simulink library "motohawk_engine_motoshare_lib"  (Simulink 6.3)
undefined symbols (not defined in the file or in its folder): cast_val, IndPowerMax, lookup_group, motohawk_tex, motohawk_vardec_config_group, motohawk_vardec_path, SampleTime, SteadyStateECT, txtTitle, WarmUpTimeConst
libraries: MotoHawk_lib x211, motohawk_control_primitives_lib x20, motohawk_annotations_lib x7, motohawk_engine_lib x5, AutoDoc_lib x4, motohawk_control_primitives_lib_new x3, motohawk_control_primitives_motoshare_lib x2
(part 1 of 7)
settings Model: Creator=Blake Suhre  LastModifiedBy=Jason_Tartt  StrictBusMsg=None

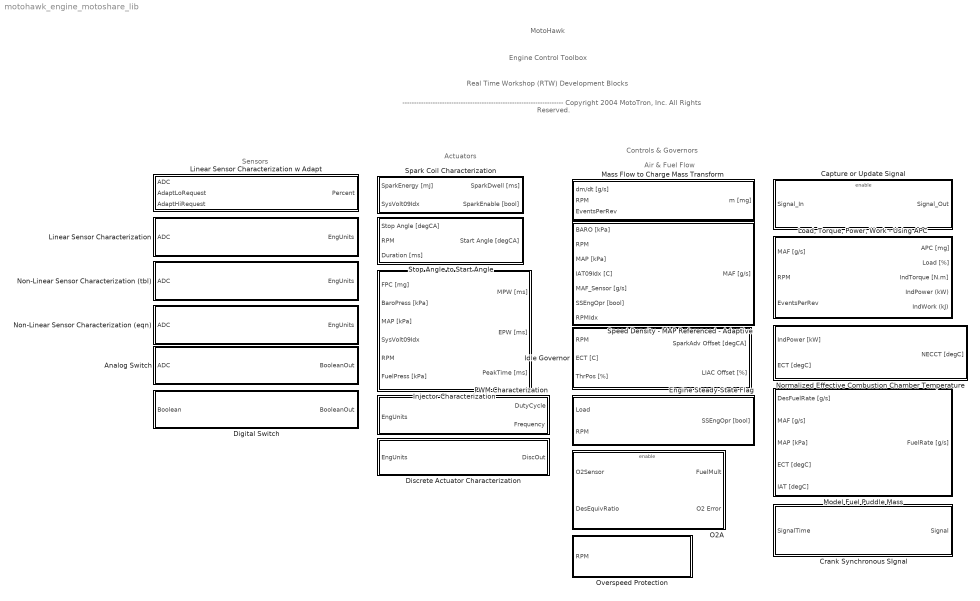
== system motohawk_engine_motoshare_lib ==
  note: Sensors
  note: MotoHawk
  note: ---------------------------------------------------------------------
      | Copyright 2004 MotoTron, Inc.  All Rights Reserved.
  note: Real Time Workshop (RTW)
      | Development Blocks
  note: Engine Control Toolbox
  note: Actuators
  note: Air & Fuel Flow
  note: Controls & Governors
  Analog Switch : Subsystem  mask(Analog Switch Characterization){prefix='ACRequest', nam='ACRequest', units='bool', polarity=High-True, parent_group='Sensors'}
      mask prompts: nam "Name"; parent_group "MotoTune Group"
      mask help:
      | This characterization block is used when digital switch behavior is used on an anolg input pin on the module.  This block inludes a calibratable threshold on the input ADC to convert that signal into a boolean signal.
      |
      | There are additional provisions to calibrate the polarity of the input and apply de-bounce delays to the switching.
      mask init:
      | lbl = ['Analog Switch: ' nam ' [' units ']'];
      | group = [parent_group ' | ' nam];
      mask StyleString: edit,edit,edit,popup(High-True|Low-True),edit
      mask Display:
      | patch([0 0 1 1], [0 0.075 0.075 0], [230/255 0/255 0/255])
      | patch([0 0 1 1], [0.025 0.05 0.05 0.025], [150/255 0/255 0/255])
      | patch([0 0 1 1], [0 0.025 0.025 0], [0/255 0/255 0/255])
      | 
      | disp(lbl);
  Capture or Update Signal : Subsystem  mask(Capture Signal At Startup){nam='Baro', count=5, units='kPa', grp='Engine Control | Run | Airflow'}
      mask prompts: nam "Signal Name"; count "Number Of Samples To Average"; grp "MotoTune GroupString Name"
      mask init:
      | lbl = sprintf('LATCH SIGNAL\nAverage of %d Samples', count);
      mask Display:
      | patch([0 0 1 1], [0 0.075 0.075 0], [230/255 0/255 0/255])
      | patch([0 0 1 1], [0.025 0.05 0.05 0.025], [150/255 0/255 0/255])
      | patch([0 0 1 1], [0 0.025 0.025 0], [0/255 0/255 0/255])
      | 
      | disp(lbl);
  Crank Synchronous SIgnal : Subsystem
      mask Type: Crank Based Sensor Value
      mask Description: This subsystem averages input signal captured at 0 and 360 degrees.
      mask Display:
      | patch([0 0 1 1], [0 0.075 0.075 0], [230/255 0/255 0/255])
      | patch([0 0 1 1], [0.025 0.05 0.05 0.025], [150/255 0/255 0/255])
      | patch([0 0 1 1], [0 0.025 0.025 0], [0/255 0/255 0/255])
      | 
      | disp('CRANK SYNCHRONOUS \nSIGNAL')
  Digital Switch : Subsystem  mask(Digital Switch Characterization){prefix='BrakeRequest', nam='BrakeRequest', units='bool', polarity=High-True, parent_group='Sensors'}
      mask prompts: nam "Name"; parent_group "MotoTune Group"
      mask help:
      | This characterization block is used when digital switch behavior is used on a digital input pin on the module.
      |
      | There are additional provisions to calibrate the polarity of the input and apply de-bounce delays to the switching.
      mask init:
      | lbl = ['Digital Switch: ' nam ' [' units ']'];
      | group = [parent_group ' | ' nam];
      mask StyleString: edit,edit,edit,popup(High-True|Low-True),edit
      mask Display:
      | patch([0 0 1 1], [0 0.075 0.075 0], [230/255 0/255 0/255])
      | patch([0 0 1 1], [0.025 0.05 0.05 0.025], [150/255 0/255 0/255])
      | patch([0 0 1 1], [0 0.025 0.025 0], [0/255 0/255 0/255])
      | 
      | disp(lbl);
  Discrete Actuator Characterization : Subsystem  mask(Discrete Actuator Characterization){prefix='MIL', nam='MIL', units='bool', parent_group='Actuators', polarity=High-True}
      mask prompts: nam "Name"; parent_group "MotoTune Group"
      mask help: Provides the ability to calibrate the polarity of the output digital state before it is applied to the digital output pin.
      mask init:
      | lbl = ['Discrete Characterization:  ' nam ];
      | group = [parent_group ' | ' nam];
      mask StyleString: edit,edit,edit,edit,popup(High-True|Low-True)
      mask Display:
      | patch([0 0 1 1], [0 0.075 0.075 0], [230/255 0/255 0/255])
      | patch([0 0 1 1], [0.025 0.05 0.05 0.025], [150/255 0/255 0/255])
      | patch([0 0 1 1], [0 0.025 0.025 0], [0/255 0/255 0/255])
      | 
      | disp(lbl);
  Engine Steady-State Flag : Subsystem  Description=|  mask(Steady-State Engine Operation){samp_time=SampleTime, group='Engine Control | States | States Config'}
      | /* Name: SSTorqueFilterConst Unit:sec ClassID:VAR StorageID:FLASH Access:RW4+RW3+NA2+NA1 TypeID:UINT2            
      |    Gain:0.001 Min:0.00 Max:65.54 Format:4.2 UpdateID:REMOTE Group:"Engine Control | States" Help:"First-order "  
      |    "filter time constant used to filter torque. This value must be less than SSTorqueTol from unfiltered torque "
      |    "before the steady-state flag can be enabled." VardecSig:6C */                                                
      |                                                                                                                  
      | /* Name: SSRPMFilterConst Unit:sec ClassID:VAR StorageID:FLASH Access:RW4+RW3+NA2+NA1 TypeID:UINT2               
      |    Gain:0.001 Min:0.00 Max:65.54 Format:4.2 UpdateID:REMOTE Group:"Engine Control | States" Help:"First-order "  
      |    "filter time constant used to filter torque. This value must be less than SSRPMTol from unfiltered torque "   
      |    "before the steady-state flag can be enabled." VardecSig:6C */                                                
      |                                                                                                                  
      | /* Name: SSTorqueTol Unit:N.m ClassID:VAR StorageID:FLASH Access:RW4+RW3+NA2+NA1 TypeID:UINT2 Gain:0.001         
      |    Min:0.00 Max:65.54 Format:4.2 UpdateID:REMOTE Group:"Engine Control | States" Help:"Tolerance within which "  
      |    "the difference between filtered and unfiltered torque must lie before the steady-state flag can be "         
      |    "enabled." VardecSig:6C */                                                                                    
      |                                                                                                                  
      | /* Name: SSRPMTol Unit:RPM ClassID:VAR StorageID:FLASH Access:RW4+RW3+NA2+NA1 TypeID:UINT2 Gain:0.01             
      |    Min:0.00 Max:655.35 Format:4.2 UpdateID:REMOTE Group:"Engine Control | States" Help:"Tolerance within which " 
      |    "the difference between filtered and unfiltered RPM must lie before the steady-state flag can be enabled."    
      |    VardecSig:6C */
      mask prompts: samp_time "Sample Time [s]:"; group "MotoTune Group String"
      mask help:
      | This block determines whether or not the engine has achieved steady-state operation. It accomplishes this by applying a first-order low-pass filter to the indicated torque and RPM inputs. The filetrcoeficeints are individually calibratable for each. Once both the filtered torque and RPM values are within the calibratable toleraance of the input values, engine operation is assumed to be steady-state.
      |
      | If 'Sample Time' is -1, then extra code and RAM will be generated to dynamically calculate dt.
      mask Display:
      | patch([0 0 1 1], [0 0.075 0.075 0], [230/255 0/255 0/255])
      | patch([0 0 1 1], [0.025 0.05 0.05 0.025], [150/255 0/255 0/255])
      | patch([0 0 1 1], [0 0.025 0.025 0], [0/255 0/255 0/255])
      | 
      | disp('ENGINE\nSTEADY-STATE\nDETERMINATION')
  Idle Governor : Subsystem
      mask Display:
      | patch([0 0 1 1], 0.5*[0 0.075 0.075 0], [230/255 0/255 0/255])
      | patch([0 0 1 1], 0.5*[0.025 0.05 0.05 0.025], [150/255 0/255 0/255])
      | patch([0 0 1 1], 0.5*[0 0.025 0.025 0], [0/255 0/255 0/255])
      | 
      | disp('IDLE GOVERNOR');
  Injector Characterization : Subsystem  Description=|
      | /* Name: InjGain Unit:ms/mg ClassID:VAR StorageID:FLASH Access:RW4+RW3+NA2+NA1 TypeID:UINT2 Gain:0.0001       
      |    Min:0.0000 Max:6.5500 Format:5.4 UpdateID:REMOTE Group:"Actuators | Injectors | Config" Help:"Gain valued "
      |    "used in the linear transformation of FPC to mechanical pulsewidth." VardecSig:6C */                       
      |                                                                                                               
      | /* Name: InjOfst Unit:ms ClassID:VAR StorageID:FLASH Access:RW4+RW3+NA2+NA1 TypeID:SINT2 Gain:0.0001          
      |    Min:-3.2768 Max:3.2767 Format:5.4 UpdateID:REMOTE Group:"Actuators | Injectors | Config" Help:"Offset "    
      |    "valued used in the linear transformation of FPC to mechanical pulsewidth." VardecSig:6C */                
      |                                                                                                               
      | /* Name: SysVolt10IdxArr Unit:volt ClassID:ORDARR StorageID:FLASH Access:RW4+RW3+NA2+NA1 TypeID:UINT1         
      |    Gain:0.1 Min:0.00 Max:25.50 Format:4.2 UpdateID:REMOTE OrdLen:10 Group:"Global Index Arrays | Voltage"     
      |    Help:"Ten breakpoint system voltage index array." VardecSig:6C */                                          
      |                                                                                                               
      | /* Name: InjTurnOnTbl Unit:ms ClassID:TBL StorageID:FLASH Access:RW4+RW3+NA2+NA1 TypeID:UINT2 Gain:0.001      
      |    Min:0.0000 Max:65.5350 Format:5.4 UpdateID:REMOTE OrdArr:SysVolt10IdxArr Group:"Actuators | Injectors"     
      |    Help:"Injector turn on time as a function of system voltage." VardecSig:6C */                              
      |                                                                                                               
      | /* Name: InjDeltaPress10IdxArr Unit:kPa ClassID:ORDARR StorageID:FLASH Access:RW4+RW3+NA2+NA1 TypeID:UINT2    
      |    Gain:0.1 Min:0.0 Max:6553.0 Format:5.1 UpdateID:REMOTE OrdLen:10 Group:"Actuators | Injectors" Help:"Ten " 
      |    "breakpoint fuel delta pressure index array." VardecSig:6C */                                              
      |                                                                                                               
      | /* Name: FueldPCompTbl Unit:kPa ClassID:TBL StorageID:FLASH Access:RW4+RW3+NA2+NA1 TypeID:UINT2 Gain:0.1      
      |    Min:0.0 Max:6553.0 Format:5.1 UpdateID:REMOTE OrdArr:InjDeltaPress10IdxArr Group:"Actuators | Injectors"   
      |    Help:"Injector delta pressure compensation table." VardecSig:6C */                                         
      |                                                                                                               
      | /* Name: InjTurnOffTbl Unit:ms ClassID:TBL StorageID:FLASH Access:RW4+RW3+NA2+NA1 TypeID:UINT2                
      |    Gain:0.01 Min:0.00 Max:655.00 Format:5.2 UpdateID:REMOTE OrdArr:InjDeltaPress10IdxArr Group:"Actuators | " 
      |    "Injectors" Help:"Injector turn off time table." VardecSig:6C */                                           
      |                                                                                                               
      | /* Name: InjMPW Unit:ms ClassID:VAR StorageID:RAM Access:RO4+RO3+NA2+NA1 TypeID:UINT2 Gain:0.01 Min:0.00      
      |    Max:655.35 Format:5.2 UpdateID:BACKGND Group:"Actuators | Injectors" Help:"Injector mechanical pulse "     
      |    "width." VardecSig:6C */                                                                                   
      |                                                                                                               
      | /* Name: InjEPW Unit:ms ClassID:VAR StorageID:RAM Access:RO4+RO3+NA2+NA1 TypeID:UINT2 Gain:0.01 Min:0.00      
      |    Max:655.35 Format:5.2 UpdateID:BACKGND Group:"Actuators | Injectors" Help:"Injector electrical pulse "     
      |    "width." VardecSig:6C */                                                                                   
      |                                                                                                               
      | /* Name: InjDeltaPress Unit:kPa ClassID:VAR StorageID:RAM Access:RO4+RO3+NA2+NA1 TypeID:UINT2 Gain:0.01       
      |    Min:0.00 Max:655.35 Format:5.2 UpdateID:BACKGND Group:"Actuators | Injectors" Help:"Delta pressure across "
      |    "the injector." VardecSig:6C */                                                                            
      | /* Name: FuelFlowCompMap Unit:mult ClassID:MAP StorageID:RAM Access:RO4+RO3+NA2+NA1 TypeID:UINT2              
      |    Gain:0.0001 Min:0.0000 Max:2.0000 Format:5.4 UpdateID:BACKGND XOrdArr:IndTorque10IdxArr YOrdArr:RPM10IdxArr
      |    Group:"Actuators | Injectors" Help:"Correction for injector fuel flow differences between injector test "  
      |    "bench and engine operating in the conditions. This map should only be calibrated after volumetric "       
      |    "efficiency has been calibrated to a reference airflow measurement device." VardecSig:6C */
      mask Description: Injector characterization block.
      mask Help: Converts the calculated fuel charge mass (FPC) value to the required electrical pulsewidth. Requires gain, offset, turn-on time vs. voltage, turn-off time vs. injector delta pressure and delta pressure pulsewidth compensation. A choice of five different injector delta pressure calculation methods are offered.
      mask Display:
      | patch([0 0 1 1], [0 0.075 0.075 0], [230/255 0/255 0/255])
      | patch([0 0 1 1], [0.025 0.05 0.05 0.025], [150/255 0/255 0/255])
      | patch([0 0 1 1], [0 0.025 0.025 0], [0/255 0/255 0/255])
      | 
      | disp('Injector\nCharacterization')
  Linear Sensor Characterization : Subsystem  mask(Linear Sensor Characterization){nam='MAP', prefix='MAP', units='kPa', inputunits=ADC, samp_time=SampleTime, parent_group='Sensors'}
      mask prompts: nam "Name"; units "Output Units"; inputunits "Input Units"; samp_time "Sample Time"; parent_group "MotoTune Group"
      mask help:
      | Converts from A/D Counts to Engineering Units, using a Gain and Offset.
      | Saturates the converted value around Min and Max values, and triggers a Fault when out of range.
      mask init:
      | lbl = ['Linear Sensor: ' nam ' [' units ']'];
      | group = [parent_group ' | ' nam];
      settings: RTWSystemCode=Function  RTWFcnNameOpts=Use subsystem name  RTWFileNameOpts=Use function name
      mask Display:
      | patch([0 0 1 1], [0 0.075 0.075 0], [230/255 0/255 0/255])
      | patch([0 0 1 1], [0.025 0.05 0.05 0.025], [150/255 0/255 0/255])
      | patch([0 0 1 1], [0 0.025 0.025 0], [0/255 0/255 0/255])
      | 
      | disp(lbl);
  Linear Sensor Characterization w Adapt : Subsystem  mask(Potentiometer Characterization with adapting endpoints.){nam='TPS', prefix='TPS', samp_time=.005, parent_group='Sensors | TPS'}
      mask prompts: nam "Name"; samp_time "Sample Time"; parent_group "MotoTune Group"
      mask help:
      | This block transforms the input from a potentiometer into a percentage, refering to the percentage of travel within the scale.
      |
      | The endpoints of the scale will adapt based on the values that block sees on the input.
      mask init:
      | lbl = ['Linear Sensor: ' nam ' [%]'];
      | lbl2 = ['With Adaption'];
      | group = [parent_group ' | ' nam];
      | units = '%';
      mask Display:
      | patch([0 0 1 1], [0 0.075 0.075 0], [230/255 0/255 0/255])
      | patch([0 0 1 1], [0.025 0.05 0.05 0.025], [150/255 0/255 0/255])
      | patch([0 0 1 1], [0 0.025 0.025 0], [0/255 0/255 0/255])
      | 
      | 
      | 
      | text(0.6,0.60,lbl,'horizontalAlignment','center');
      | text(0.6,0.30,lbl2,'horizontalAlignment','center');
  "Load, Torque, Power, Work - Using APC" : Subsystem
      mask Display:
      | patch([0 0 1 1], 0.8*[0 0.075 0.075 0], [230/255 0/255 0/255])
      | patch([0 0 1 1], 0.8*[0.025 0.05 0.05 0.025], [150/255 0/255 0/255])
      | patch([0 0 1 1], 0.8*[0 0.025 0.025 0], [0/255 0/255 0/255])
      | 
      | disp('LOAD, TORQUE,\nPOWER, AND WORK\nCOMPUTATION\nUSING APC');
  Mass Flow to Charge Mass Transform : Subsystem
      mask Description: Converts mass flow rate to the equivalent per cylinder charge mass.
      mask Help:
      | Given the mass flow rate [g/s], RPM and the total number of combustion events per crankshaft revolution, this block calculates the equivalent charge mass ingested per cylinder.
      | 
      | Note: as an example, the number of cylinder events per revolution would be 2 for a four cylinder four-stroke engine and 4 for a four-cylinder two-stroke engine.
      mask Display:
      | patch([0 0 1 1], [0 0.075 0.075 0], [230/255 0/255 0/255])
      | patch([0 0 1 1], [0.025 0.05 0.05 0.025], [150/255 0/255 0/255])
      | patch([0 0 1 1], [0 0.025 0.025 0], [0/255 0/255 0/255])
      | 
      | disp('MASS FLOW\nTO CHARGE MASS\nTRANSFORM')
  Model Fuel Puddle Mass : Subsystem  mask{group_cal='Engine Control | Run | Fuel | Transient Fuel', group_dis='Engine Control | Run | Fuel | Transient Fuel'}
      mask prompts: group_cal "MotoTune Calibration Group String"; group_dis "MotoTune Display Group String"
      mask Display:
      | patch([0 0 1 1], 0.5*[0 0.075 0.075 0], [230/255 0/255 0/255])
      | patch([0 0 1 1], 0.5*[0.025 0.05 0.05 0.025], [150/255 0/255 0/255])
      | patch([0 0 1 1], 0.5*[0 0.025 0.025 0], [0/255 0/255 0/255])
      | 
      | disp('TAU-X\nTRANSIENT\nFUELING');
  Non-Linear Sensor Characterization (eqn) : Subsystem  mask(Non-Linear Sensor Characterization (eqn)){nam='ECT', prefix='ECT', units='C', inputunits='ADC', numcoef=6, samp_time=SampleTime, parent_group='Sensors'}
      mask prompts: nam "Name"; units "Output Units"; inputunits "Input Units"; numcoef "Number Of Coefficients"; samp_time "Sample Time"; parent_group "MotoTune Group"
      mask help:
      | Converts from A/D Counts to Engineering Units using a calibration polynomial.
      | Saturates the converted value around Min and Max values and triggers a Fault when out of range.
      mask init:
      | lbl = ['Non-Linear Sensor (eqn): ' nam ' [' units ']'];
      | group = [parent_group ' | ' nam];
      settings: RTWSystemCode=Function  RTWFcnNameOpts=Use subsystem name  RTWFileNameOpts=Use function name
      mask Display:
      | patch([0 0 1 1], [0 0.075 0.075 0], [230/255 0/255 0/255])
      | patch([0 0 1 1], [0.025 0.05 0.05 0.025], [150/255 0/255 0/255])
      | patch([0 0 1 1], [0 0.025 0.025 0], [0/255 0/255 0/255])
      | 
      | disp(lbl);
  Non-Linear Sensor Characterization (tbl) : Subsystem  mask(Non-Linear Sensor Characterization (tbl)){nam='IAT', prefix='IAT', units='C', inputunits='ADC', tblsize=20, samp_time=SampleTime, parent_group='Sensors'}
      mask prompts: nam "Name"; units "Output Units"; inputunits "Input Units"; tblsize "Table Size"; samp_time "Sample Time"; parent_group "MotoTune Group"
      mask help:
      | Converts from A/D Counts to Engineering Units using a 1-D Table Lookup.
      | Saturates the converted value around Min and Max values and triggers a Fault when out of range.
      mask init:
      | lbl = ['Non-Linear Sensor (tbl): ' nam ' [' units ']'];
      | group = [parent_group ' | ' nam];
      settings: RTWSystemCode=Function  RTWFcnNameOpts=Use subsystem name  RTWFileNameOpts=Use function name
      mask Display:
      | patch([0 0 1 1], [0 0.075 0.075 0], [230/255 0/255 0/255])
      | patch([0 0 1 1], [0.025 0.05 0.05 0.025], [150/255 0/255 0/255])
      | patch([0 0 1 1], [0 0.025 0.025 0], [0/255 0/255 0/255])
      | 
      | disp(lbl);
  Normalized Effective Combustion Chamber Temperature : Subsystem  Description=|  mask(Steady-State Engine Operatio){}
      | /* Name: SSTorqueFilterConst Unit:sec ClassID:VAR StorageID:FLASH Access:RW4+RW3+NA2+NA1 TypeID:UINT2            
      |    Gain:0.001 Min:0.00 Max:65.54 Format:4.2 UpdateID:REMOTE Group:"Engine Control | States" Help:"First-order "  
      |    "filter time constant used to filter torque. This value must be less than SSTorqueTol from unfiltered torque "
      |    "before the steady-state flag can be enabled." VardecSig:6C */                                                
      |                                                                                                                  
      | /* Name: SSRPMFilterConst Unit:sec ClassID:VAR StorageID:FLASH Access:RW4+RW3+NA2+NA1 TypeID:UINT2               
      |    Gain:0.001 Min:0.00 Max:65.54 Format:4.2 UpdateID:REMOTE Group:"Engine Control | States" Help:"First-order "  
      |    "filter time constant used to filter torque. This value must be less than SSRPMTol from unfiltered torque "   
      |    "before the steady-state flag can be enabled." VardecSig:6C */                                                
      |                                                                                                                  
      | /* Name: SSTorqueTol Unit:N.m ClassID:VAR StorageID:FLASH Access:RW4+RW3+NA2+NA1 TypeID:UINT2 Gain:0.001         
      |    Min:0.00 Max:65.54 Format:4.2 UpdateID:REMOTE Group:"Engine Control | States" Help:"Tolerance within which "  
      |    "the difference between filtered and unfiltered torque must lie before the steady-state flag can be "         
      |    "enabled." VardecSig:6C */                                                                                    
      |                                                                                                                  
      | /* Name: SSRPMTol Unit:RPM ClassID:VAR StorageID:FLASH Access:RW4+RW3+NA2+NA1 TypeID:UINT2 Gain:0.01             
      |    Min:0.00 Max:655.35 Format:4.2 UpdateID:REMOTE Group:"Engine Control | States" Help:"Tolerance within which " 
      |    "the difference between filtered and unfiltered RPM must lie before the steady-state flag can be enabled."    
      |    VardecSig:6C */
      mask Display:
      | patch([0 0 1 1], [0 0.075 0.075 0], [230/255 0/255 0/255])
      | patch([0 0 1 1], [0.025 0.05 0.05 0.025], [150/255 0/255 0/255])
      | patch([0 0 1 1], [0 0.025 0.025 0], [0/255 0/255 0/255])
      | 
      | disp('COMBUSTION CHAMBER\nTEMPERATURE');
  O2A : Subsystem  TreatAsAtomicUnit=on  mask(Closed-Loop O2 Control){bank=A, display_group=lookup_group(gcb, 'O2Display'), cal_group=lookup_group(gcb, 'O2BankA')}
      mask prompts: display_group "MotoTune Display Group"; cal_group "MotoTune Calibration Group"
      mask StyleString: popup(A|B),edit,edit
      mask Display:
      | patch([0 0 1 1], 0.5*[0 0.075 0.075 0], [230/255 0/255 0/255])
      | patch([0 0 1 1], 0.5*[0.025 0.05 0.05 0.025], [150/255 0/255 0/255])
      | patch([0 0 1 1], 0.5*[0 0.025 0.025 0], [0/255 0/255 0/255])
      | 
      | disp(['O2 Control\nBank ' bank]);
  Overspeed Protection : Subsystem
      mask Description:
      | Block allows for three levels of overspeed rev limits, and will set three fault accordingly.
      | 
      | Soft Overspeed, Medium Overspeed, and Hard Overspeed.
      mask Display:
      | patch([0 0 1 1], 0.5*[0 0.075 0.075 0], [230/255 0/255 0/255])
      | patch([0 0 1 1], 0.5*[0.025 0.05 0.05 0.025], [150/255 0/255 0/255])
      | patch([0 0 1 1], 0.5*[0 0.025 0.025 0], [0/255 0/255 0/255])
      | 
      | disp('RPM LIMITER');
  PWM Characterization : Subsystem  mask(Linear Actuator Characterization){nam='LIAC', prefix='LIAC_', units='%', parent_group=motohawk_vardec_path(gcb)}
      mask prompts: nam "Name"; parent_group "MotoTune Group"
      mask help:
      | Scales the duty cycle of a PWM signal using a Gain and Offset with a calibratable PWM Frequency.
      | Saturates the converted value around Min and Max values, and converts the signal to the appropriate fixed-point format for use with motoHawk PWM blocks.
      mask init:
      | lbl = ['PWM Characterization: ' nam ];
      | group = [parent_group ' | ' nam];
      settings: RTWSystemCode=Function  RTWFcnNameOpts=Use subsystem name  RTWFileNameOpts=Use function name
      mask Display:
      | patch([0 0 1 1], [0 0.075 0.075 0], [230/255 0/255 0/255])
      | patch([0 0 1 1], [0.025 0.05 0.05 0.025], [150/255 0/255 0/255])
      | patch([0 0 1 1], [0 0.025 0.025 0], [0/255 0/255 0/255])
      | 
      | disp(lbl);
  Spark Coil Characterization : Subsystem  Description=|  mask{group='Actuators | Coils'}
      | /* Name: CoilDrvrDlyTime Unit:us ClassID:VAR StorageID:FLASH Access:RW4+RW3+NA2+NA1 TypeID:UINT2 Gain:0.1       
      |    Min:0.00 Max:6553.50 Format:6.2 UpdateID:REMOTE Group:"Actuators | Coils" Help:"Coil driver delay time "     
      |    "between initiation of the EST signal and the initiation of coil dwell." VardecSig:6C */                     
      |                                                                                                                 
      | /* Name: SysVolt10IdxArr Unit:volt ClassID:VAR StorageID:FLASH Access:RW4+RW3+NA2+NA1 TypeID:UINT1 Gain:0.1     
      |    Min:0.00 Max:25.50 Format:4.2 UpdateID:REMOTE Group:"Global Index Arrays | Voltage" Help:"Ten breakpoint "   
      |    "system voltage index array." VardecSig:6C */                                                                
      |                                                                                                                 
      | /* Name: SpkEnergy10IdxArr Unit:volt ClassID:VAR StorageID:FLASH Access:RW4+RW3+NA2+NA1 TypeID:UINT1            
      |    Gain:0.1 Min:0.00 Max:25.50 Format:4.2 UpdateID:REMOTE Group:"Actuators | Coils" Help:"Ten breakpoint spark "
      |    "energy index array." VardecSig:6C */                                                                        
      |                                                                                                                 
      | /* Name: CoilDwellMap Unit:ms ClassID:MAP StorageID:FLASH Access:RW4+RW3+NA2+NA1 TypeID:UINT2 Gain:0.01         
      |    Min:0.00 Max:655.35 Format:4.2 UpdateID:REMOTE XOrdArr:SpkEnergy10IdxArr YOrdArr:SysVolt10IdxArr             
      |    Group:"Actuators | Coils" Help:"Required coil dwell map as a function of system voltage and spark energy."   
      |    VardecSig:6C */
      mask prompts: group "MotoTune Group String"
      mask help: Coil characterization block.
      mask Help: Given the desired spark energy and system voltage, this block determines the required coil dwell period. Requires calibration of the dwell map and the delay time.
      mask Display:
      | patch([0 0 1 1], [0 0.075 0.075 0], [230/255 0/255 0/255])
      | patch([0 0 1 1], [0.025 0.05 0.05 0.025], [150/255 0/255 0/255])
      | patch([0 0 1 1], [0 0.025 0.025 0], [0/255 0/255 0/255])
      | 
      | disp('COIL\nCHRZN.')
  Speed Density - MAP Referenced - Adaptive : Subsystem  Description=|
      | /* Name: PortPressRatio20IdxArr Unit:unitless ClassID:ORDARR StorageID:FLASH Access:RW4+RW3+NA2+NA1              
      |    TypeID:UINT2 Gain:0.0001 Min:0.0000 Max:6.5535 Format:5.4 UpdateID:REMOTE OrdLen:20 Group:"Engine Control | " 
      |    "Run | Airflow" Help:"Port pressure ratio index array. Used for speed-density flow computations." VardecSig:6E
      |    */                                                                                                            
      |                                                                                                                  
      | /* Name: RPM20IdxArr Unit:RPM20IdxArr ClassID:ORDARR StorageID:FLASH Access:RW4+RW3+NA2+NA1                      
      |    TypeID:UINT2 Gain:0.1 Min:0.0 Max:6553.0 Format:5.1 UpdateID:REMOTE OrdLen:20 Group:"Global "                 
      |    "Index Arrays | RPM" Help:"20 breakpoint RPM index array." VardecSig:5E */                                    
      |                                                                                                                  
      | /* Name: VolEffMap Unit:Unitless ClassID:MAP StorageID:FLASH Access:RW4+RW3+NA2+NA1 TypeID:UINT2                 
      |    Gain:0.0001 Min:0.00 Max:6.55 Format:6.2 UpdateID:REMOTE XOrdArr:PortPressRatio20IdxArr                       
      |    YOrdArr:RPM20IdxArr Group:"Engine Control | Run | Airflow" Help:"Engine volumetric efficency "                
      |    "map." VardecSig:61 */                                                                                        
      |                                                                                                                  
      | /* Name: IAT10IdxArr Unit:C ClassID:ORDARR StorageID:FLASH Access:RW4+RW3+NA2+NA1                                
      |    TypeID:SINT2 Gain:0.01 Min:-327.6800 Max:327.6700 Format:5.4 UpdateID:REMOTE OrdLen:10                        
      |    Group:"Engine Control | Run | Airflow" Help:"10 breakpoint intake air temperture index "                      
      |    "array." VardecSig:5C */                                                                                      
      |                                                                                                                  
      | /* Name: VETempCorrTbl ClassID:TBL StorageID:FLASH Access:RW4+RW3+NA2+NA1 TypeID:UINT2 Gain:0.0001 Min:0.00      
      |    Max:6.55 Format:4.2 UpdateID:REMOTE OrdArr:IAT10IdxArr Group:"Engine Control | Run | Airflow"                 
      |    Help:"Volumetric efficiency temperature correction table." VardecSig:6C */                                    
      |                                                                                                                  
      | /* Name: BaroPress10IdxArr Unit:C ClassID:ORDARR StorageID:FLASH Access:RW4+RW3+NA2+NA1                          
      |    TypeID:UINT2 Gain:0.01 Min:0.0000 Max:655.3500 Format:5.4 UpdateID:REMOTE OrdLen:10                           
      |    Group:"Engine Control | Run | Airflow" Help:"10 breakpoint barometric pressure index "                        
      |    "array." VardecSig:5C */                                                                                      
      |                                                                                                                  
      | /* Name: VEBaroCorrTbl ClassID:TBL StorageID:FLASH Access:RW4+RW3+NA2+NA1 TypeID:UINT2 Gain:0.0001 Min:0.00      
      |    Max:6.55 Format:4.2 UpdateID:REMOTE OrdArr:BaroPress10IdxArr Group:"Engine Control | Run | Airflow"           
      |    Help:"Volumetric efficiency barometric pressure correction table." VardecSig:6C */                            
      |                                                                                                                  
      | /* Name: CylSweptVol Unit:cm^3 ClassID:VAR StorageID:FLASH Access:RW4+RW3+NA2+NA1 TypeID:UINT2 Gain:0.1          
      |    Min:0.0 Max:6553.0 Format:5.1 UpdateID:REMOTE Group:"Engine Control | Run | Airflow" Help:"Cylinder swept "   
      |    "volume." VardecSig:6C */                                                                                     
      |                                                                                                                  
      | /* Name: MAFPort Unit:g/s ClassID:VAR StorageID:RAM Access:RO4+RO3+NA2+NA1 TypeID:UINT2 Gain:0.01                
      |    Min:0.00 Max:655.00 Format:5.2 UpdateID:BACKGND Group:"Engine Control | Run | Airflow" Help:"Total "          
      |    "ingested cylinder charge mass flow rate. The sum of all port flows. This values includes any EGR and "       
      |    "Purge mass flows." VardecSig:6A */                                                                           
      |                                                                                                                  
      | /* Name: CombEventsPerRev ClassID:VAR StorageID:FLASH Access:RW4+RW3+NA2+NA1 TypeID:UINT1 Gain:0.5 Min:0.5       
      |    Max:127.0 Format:4.1 UpdateID:REMOTE Group:"Engine Control | Run | Airflow" Help:"Number of conbustion "      
      |    "events per engine revolution. For example, for a four-stroke, eight cylinder engine the value would be 4."   
      |    VardecSig:6C */
      mask Description: Calculates air mass flow rate per cylinder. The estimated mass flow rate is that of the entire mixture: air, EGR and purge.
      mask Help: Given calibrations for the volumetric efficiency map, cylinder swept volume [cm3] and the VE temperature and pressure correction tables, the block calculates the air mass flow rate [g/s] per cylinder, given the barometric and manifold pressures [kPa], the manifold air temperature [C] and RPM.
      mask Display:
      | patch([0 0 1 1], 0.5*[0 0.075 0.075 0], [230/255 0/255 0/255])
      | patch([0 0 1 1], 0.5*[0.025 0.05 0.05 0.025], [150/255 0/255 0/255])
      | patch([0 0 1 1], 0.5*[0 0.025 0.025 0], [0/255 0/255 0/255])
      | 
      | disp('MAP-REFERENCED\nSPEED-DENSITY\nCOMPUTATION\n(adaptive)');
  Stop Angle to Start Angle : Subsystem  Description=|
      | /* Name: CoilDrvrDlyTime Unit:us ClassID:VAR StorageID:FLASH Access:RW4+RW3+NA2+NA1 TypeID:UINT2 Gain:0.1       
      |    Min:0.00 Max:6553.50 Format:6.2 UpdateID:REMOTE Group:"Actuators | Coils" Help:"Coil driver delay time "     
      |    "between initiation of the EST signal and the initiation of coil dwell." VardecSig:6C */                     
      |                                                                                                                 
      | /* Name: SysVolt10IdxArr Unit:volt ClassID:VAR StorageID:FLASH Access:RW4+RW3+NA2+NA1 TypeID:UINT1 Gain:0.1     
      |    Min:0.00 Max:25.50 Format:4.2 UpdateID:REMOTE Group:"Global Index Arrays | Voltage" Help:"Ten breakpoint "   
      |    "system voltage index array." VardecSig:6C */                                                                
      |                                                                                                                 
      | /* Name: SpkEnergy10IdxArr Unit:volt ClassID:VAR StorageID:FLASH Access:RW4+RW3+NA2+NA1 TypeID:UINT1            
      |    Gain:0.1 Min:0.00 Max:25.50 Format:4.2 UpdateID:REMOTE Group:"Actuators | Coils" Help:"Ten breakpoint spark "
      |    "energy index array." VardecSig:6C */                                                                        
      |                                                                                                                 
      | /* Name: CoilDwellMap Unit:ms ClassID:MAP StorageID:FLASH Access:RW4+RW3+NA2+NA1 TypeID:UINT2 Gain:0.01         
      |    Min:0.00 Max:655.35 Format:4.2 UpdateID:REMOTE XOrdArr:SpkEnergy10IdxArr YOrdArr:SysVolt10IdxArr             
      |    Group:"Actuators | Coils" Help:"Required coil dwell map as a function of system voltage and spark energy."   
      |    VardecSig:6C */
      mask Type: Stop Angle to Start Angle
      mask Description: Stop Angle to Start Angle calculation.  Subtracts the duration of a Pulse Width in the angle domain from a given Stop Angle.
      mask Display:
      | patch([0 0 1 1], [0 0.075 0.075 0], [230/255 0/255 0/255])
      | patch([0 0 1 1], [0.025 0.05 0.05 0.025], [150/255 0/255 0/255])
      | patch([0 0 1 1], [0 0.025 0.025 0], [0/255 0/255 0/255])

== system motohawk_engine_motoshare_lib/Analog Switch ==
  ADC : Inport
  0 = No Inversion 1 = Inversion : MotoHawk_lib/Calibration & Probing Blocks/motohawk_calibration  nam=[prefix 'Polarity']  val=boolean(polarity-1)  storage=Calibration  show_more=on  name_source=Use Parameter  data_type=Inherit from 'Default Value'  read_level=1  write_level=1  ovr_cals=on  view_as=Number  enum_struct={'Disabled', 'Enabled'}  vector_style=Wide Row  use_help_units=on  help="'0 = High True    1 = Low True'"  units='bool'  use_header_enum=off  row_header_enum={}  col_header_enum={}  use_min_max=off  min_val=-inf  max_val=inf  use_precision=off  precision=''  gain=1  offset=0  exp=1  use_mototune_group=on  mototune_group=[group ' | ' nam ' | ' nam ' Config']
  Data Type Conversion : DataTypeConversion  SaturateOnIntegerOverflow=on  RndMeth=Zero
  Logical Operator : Logic  Operator=XOR
  Override in Engineering Units : MotoHawk_lib/Calibration & Probing Blocks/motohawk_override_abs  parent_name=nam  show_more=on  name_source=Use Parameter  parent_read_level=1  parent_override_level=1  view_as=Number  enum_struct={'Disabled', 'Enabled'}  use_help_units=on  parent_help='Override actuator, in engineering units'  parent_units=units  use_min_max=off  parent_min=-inf  parent_max=inf  use_precision=off  parent_precision=''  parent_gain=1  parent_offset=0  parent_exp=1  use_mototune_group=on  parent_group=[group ' | ' nam]
  Relational Operator : RelationalOperator  Operator=>
  Switch Debounce : motohawk_control_primitives_motoshare_lib/Switch Debounce
  SwitchPoint : MotoHawk_lib/Calibration & Probing Blocks/motohawk_calibration  nam=[prefix 'SwitchPt']  val=switchpoint  storage=Calibration  show_more=on  name_source=Use Parameter  data_type=Inherit from 'Default Value'  read_level=1  write_level=1  ovr_cals=on  view_as=Number  enum_struct={'Disabled', 'Enabled'}  vector_style=Wide Row  use_help_units=on  help='Defines switch point in ADC units boolean conversion'  units='ADC'  use_header_enum=off  row_header_enum={}  col_header_enum={}  use_min_max=off  min_val=-inf  max_val=inf  use_precision=off  precision=''  gain=1  offset=0  exp=1  use_mototune_group=on  mototune_group=[group ' | ' nam ' Config']
  motohawk_calibration : MotoHawk_lib/Calibration & Probing Blocks/motohawk_calibration  nam=[prefix 'DebouncePeriod']  val=4.5  storage=Calibration  show_more=on  name_source=Use Parameter  data_type=Inherit from 'Default Value'  read_level=1  write_level=1  ovr_cals=on  view_as=Number  enum_struct={'Disabled', 'Enabled'}  vector_style=Wide Row  use_help_units=on  help='Debounce timer for the switch input.'  units='s'  use_header_enum=off  row_header_enum={}  col_header_enum={}  use_min_max=off  min_val=-inf  max_val=inf  use_precision=off  precision=''  gain=1  offset=0  exp=1  use_mototune_group=on  mototune_group=[group ' | ' nam ' | ' nam ' Config']
  motohawk_probe1 : MotoHawk_lib/Calibration & Probing Blocks/motohawk_probe  nam=nam  show_more=on  name_source=Use Parameter  read_level=1  view_as=Number  enum_struct={'Disabled', 'Enabled'}  vector_style=Wide Row  use_help_units=on  help='Display output in engineering units'  units=units  use_header_enum=off  row_header_enum={}  col_header_enum={}  use_precision=off  precision=''  gain=1  offset=0  exp=1  use_mototune_group=on  mototune_group=[group ' | ' nam]
  motohawk_probe2 : MotoHawk_lib/Calibration & Probing Blocks/motohawk_probe  nam=[nam '_Raw']  show_more=on  name_source=Use Parameter  read_level=1  view_as=Number  enum_struct={'Disabled', 'Enabled'}  vector_style=Wide Row  use_help_units=on  help='Display output in engineering units'  units='ADC'  use_header_enum=off  row_header_enum={}  col_header_enum={}  use_precision=off  precision=''  gain=1  offset=0  exp=1  use_mototune_group=on  mototune_group=group
  BooleanOut : Outport
  wires:
  0 = No Inversion 1 = Inversion/1 -> Logical Operator/2
  Override in Engineering Units/1 -> BooleanOut/1, motohawk_probe1/1
  Logical Operator/1 -> Switch Debounce/1
  Switch Debounce/1 -> Override in Engineering Units/1
  motohawk_calibration/1 -> Switch Debounce/2
  Data Type Conversion/1 -> motohawk_probe2/1, Relational Operator/1
  SwitchPoint/1 -> Relational Operator/2
  ADC/1 -> Data Type Conversion/1
  Relational Operator/1 -> Logical Operator/1

== system motohawk_engine_motoshare_lib/Capture or Update Signal ==
  note: Count up to "BARO_Count" samples
  Signal_In : Inport
  Enable : EnablePort
  Add : Sum  OutScaling=2^-10
  Add1 : Sum  Inputs=+-  OutScaling=2^-10
  Collect Average : Subsystem
  Constant : Constant  Value=int8(1)  SampleTime=-1
  Logical Operator : Logic  AllPortsSameDT=off  OutDataTypeMode=Boolean
  Relational Operator : RelationalOperator  Operator=<=
  Relational Operator1 : RelationalOperator  Operator=>
  Sum : Sum  Inputs=++|  InputSameDT=on
  Switch : Switch  Threshold=1  ZeroCross=off  InputSameDT=on
  TwoSampleBuffer ToIgnore : Constant  Value=2  SampleTime=-1
  Unit Delay : UnitDelay  Orientation=left  SampleTime=-1
  motohawk_calibration : MotoHawk_lib/Calibration & Probing Blocks/motohawk_calibration  nam=[nam '_Count']  val=int8(count)  storage=Calibration  show_more=on  name_source=Use Parameter  data_type=Inherit from 'Default Value'  read_level=1  write_level=1  ovr_cals=on  view_as=Number  enum_struct={'Disabled', 'Enabled'}  vector_style=Wide Row  use_help_units=on  help='Number of samples to average at key-up to produce signal value'  units=''  use_header_enum=off  row_header_enum={}  col_header_enum={}  use_min_max=off  min_val=-inf  max_val=inf  use_precision=off  precision=''  gain=1  offset=0  exp=1  use_mototune_group=on  mototune_group=grp
  motohawk_override_rel : MotoHawk_lib/Calibration & Probing Blocks/motohawk_override_rel  parent_name=nam  show_more=on  name_source=Use Parameter  parent_read_level=1  parent_override_level=1  use_help_units=on  parent_help='Provides an override to the input by adding this amount to either the locked or running value'  parent_units=units  use_min_max=off  parent_min=-inf  parent_max=inf  use_precision=off  parent_precision=''  parent_gain=1  parent_offset=0  parent_exp=1  use_mototune_group=on  parent_group=grp
  motohawk_probe : MotoHawk_lib/Calibration & Probing Blocks/motohawk_probe  nam=nam  show_more=on  name_source=Use Parameter  read_level=1  view_as=Number  enum_struct={'Disabled', 'Enabled'}  vector_style=Wide Row  use_help_units=on  help=''  units=units  use_header_enum=off  row_header_enum={}  col_header_enum={}  use_precision=off  precision=''  gain=1  offset=0  exp=1  use_mototune_group=on  mototune_group=grp
  Signal_Out : Outport
  wires:
  Add1/1 -> Collect Average/1(Count)
  Relational Operator1/1 -> Logical Operator/2
  Logical Operator/1 -> Collect Average/Enable
  TwoSampleBuffer ToIgnore/1 -> Add1/2, Relational Operator1/2, Add/2
  Add/1 -> Switch/3, Relational Operator/2
  motohawk_calibration/1 -> Add/1
  motohawk_override_rel/1 -> Signal_Out/1, motohawk_probe/1
  Constant/1 -> Sum/2
  Unit Delay/1 -> Sum/1
  Signal_In/1 -> Collect Average/2(Signal)
  Collect Average/1(Captured_Signal) -> motohawk_override_rel/1
  Switch/1 -> Add1/1, Unit Delay/1
  Relational Operator/1 -> Logical Operator/1, Switch/2
  Sum/1 -> Relational Operator1/1, Relational Operator/1, Switch/1

== system motohawk_engine_motoshare_lib/Crank Synchronous SIgnal ==
  SignalTime : Inport
  Merge : Merge
  Mux : Mux  Orientation=down  Inputs=2
  Once at Startup : Subsystem  TreatAsAtomicUnit=on
  TDC and MID_TDC : Subsystem  TreatAsAtomicUnit=on
  motohawk_trigger : MotoHawk_lib/Trigger Blocks/motohawk_trigger  Tag=Trigger  Orientation=down  trigger=FGND_TDC_EVENT  function_name=Trigger_FGND_TDC_EVENT_4167p0011  priority_order=0  inherited=off  run_disabled=off  override_app_monitor=off  target=ECU555_80
  motohawk_trigger1 : MotoHawk_lib/Trigger Blocks/motohawk_trigger  Tag=Trigger  Orientation=down  trigger=FGND_MID_TDC_EVENT  function_name=Trigger_FGND_MID_TDC_EVENT_4167p001  priority_order=0  inherited=off  run_disabled=off  override_app_monitor=off  target=ECU555_80
  motohawk_trigger2 : MotoHawk_lib/Trigger Blocks/motohawk_trigger  Tag=Trigger  Orientation=down  trigger=STARTUP_EVENT  function_name=Trigger_STARTUP_EVENT_4167p0009  priority_order=0  inherited=off  run_disabled=off  override_app_monitor=off  target=ECU555_80
  Signal : Outport
  wires:
  TDC and MID_TDC/1(Signal_Ave) -> Merge/2
  Once at Startup/1(Signal_StartUp) -> Merge/1
  Merge/1 -> Signal/1
  motohawk_trigger2/1 -> Once at Startup/Trigger
  motohawk_trigger1/1 -> Mux/2
  motohawk_trigger/1 -> Mux/1
  Mux/1 -> TDC and MID_TDC/Trigger
  SignalTime/1 -> Once at Startup/1(Signal_Time), TDC and MID_TDC/1(Signal_Time)

== system motohawk_engine_motoshare_lib/Digital Switch ==
  Boolean : Inport
  0 = No Inversion 1 = Inversion : MotoHawk_lib/Calibration & Probing Blocks/motohawk_calibration  nam=[prefix 'Polarity']  val=boolean(polarity-1)  storage=Calibration  show_more=on  name_source=Use Parameter  data_type=Inherit from 'Default Value'  read_level=1  write_level=1  ovr_cals=on  view_as=Number  enum_struct={'Disabled', 'Enabled'}  vector_style=Wide Row  use_help_units=on  help="'0 = High True    1 = Low True'"  units='bool'  use_header_enum=off  row_header_enum={}  col_header_enum={}  use_min_max=off  min_val=-inf  max_val=inf  use_precision=off  precision=''  gain=1  offset=0  exp=1  use_mototune_group=on  mototune_group=[group ' | ' nam ' | ' nam ' Config']
  Logical Operator : Logic  Operator=XOR
  Override in Engineering Units : MotoHawk_lib/Calibration & Probing Blocks/motohawk_override_abs  parent_name=nam  show_more=on  name_source=Use Parameter  parent_read_level=1  parent_override_level=1  view_as=Number  enum_struct={'Disabled', 'Enabled'}  use_help_units=on  parent_help='Override actuator, in engineering units'  parent_units=units  use_min_max=off  parent_min=-inf  parent_max=inf  use_precision=off  parent_precision=''  parent_gain=1  parent_offset=0  parent_exp=1  use_mototune_group=on  parent_group=[group ' | ' nam]
  Switch Debounce : motohawk_control_primitives_motoshare_lib/Switch Debounce
  motohawk_calibration : MotoHawk_lib/Calibration & Probing Blocks/motohawk_calibration  nam=[prefix 'DebouncePeriod']  val=4.5  storage=Calibration  show_more=on  name_source=Use Parameter  data_type=Inherit from 'Default Value'  read_level=1  write_level=1  ovr_cals=on  view_as=Number  enum_struct={'Disabled', 'Enabled'}  vector_style=Wide Row  use_help_units=on  help='Debounce timer for the switch input.'  units='s'  use_header_enum=off  row_header_enum={}  col_header_enum={}  use_min_max=off  min_val=-inf  max_val=inf  use_precision=off  precision=''  gain=1  offset=0  exp=1  use_mototune_group=on  mototune_group=[group ' | ' nam ' | ' nam ' Config']
  motohawk_probe : MotoHawk_lib/Calibration & Probing Blocks/motohawk_probe  nam=[prefix 'Raw']  show_more=on  name_source=Use Parameter  read_level=1  view_as=Number  enum_struct={'Disabled', 'Enabled'}  vector_style=Wide Row  use_help_units=on  help='Display output in engineering units'  units=units  use_header_enum=off  row_header_enum={}  col_header_enum={}  use_precision=off  precision=''  gain=1  offset=0  exp=1  use_mototune_group=on  mototune_group=[group ' | ' nam]
  motohawk_probe1 : MotoHawk_lib/Calibration & Probing Blocks/motohawk_probe  nam=nam  show_more=on  name_source=Use Parameter  read_level=1  view_as=Number  enum_struct={'Disabled', 'Enabled'}  vector_style=Wide Row  use_help_units=on  help='Display output in engineering units'  units=units  use_header_enum=off  row_header_enum={}  col_header_enum={}  use_precision=off  precision=''  gain=1  offset=0  exp=1  use_mototune_group=on  mototune_group=[group ' | ' nam]
  BooleanOut : Outport
  wires:
  motohawk_calibration/1 -> Switch Debounce/2
  Switch Debounce/1 -> Override in Engineering Units/1
  Logical Operator/1 -> Switch Debounce/1
  Override in Engineering Units/1 -> motohawk_probe1/1, BooleanOut/1
  0 = No Inversion 1 = Inversion/1 -> Logical Operator/2
  Boolean/1 -> motohawk_probe/1, Logical Operator/1
